simulink model "Simulink"  (R2023a)
settings: Solver=ode15s  StartTime=0.0  StopTime=10.0  RelTol=1e-3
settings Model: Creator=biom3  LastModifiedBy=biom3
settings DataIOCC: SaveOutput=off  SignalLogging=off  DSMLogging=off  SaveTime=off  ReturnWorkspaceOutputs=off

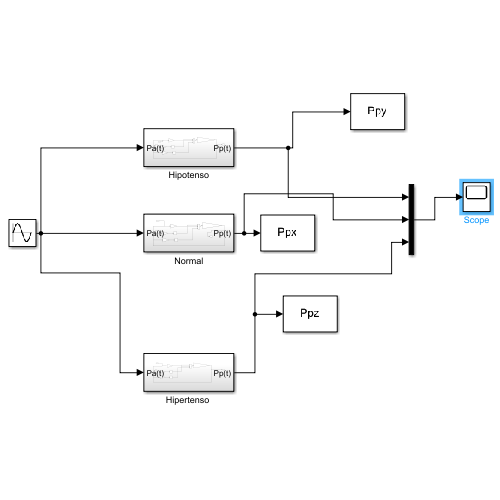
[thumbnail: Simulink's stored preview of the top-level diagram]
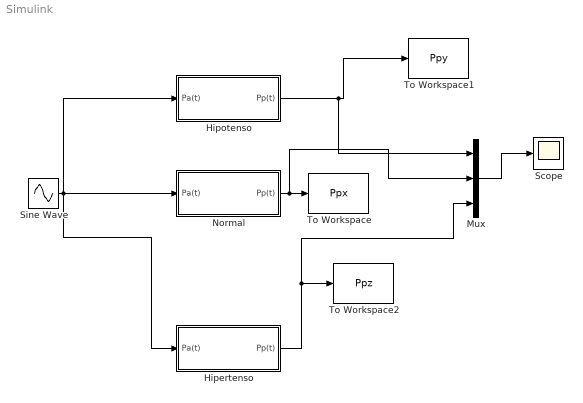
== system Simulink ==
  "Hipertenso " : Subsystem
  Hipotenso : Subsystem
  Mux : Mux  Inputs=3
  Normal : Subsystem
  Scope : Scope
  Sine Wave : Sin  Frequency=2*pi*(95/61)  SampleTime=0
  To Workspace : ToWorkspace  VariableName=Ppx  SaveFormat=Timeseries  SampleTime=-1
  To Workspace1 : ToWorkspace  VariableName=Ppy  SaveFormat=Timeseries  SampleTime=-1
  To Workspace2 : ToWorkspace  VariableName=Ppz  SaveFormat=Timeseries  SampleTime=-1
  wires:
  Mux/1 -> Scope/1
  Sine Wave/1 -> Hipotenso/1(Pa(t)), Normal/1(Pa(t)), "Hipertenso "/1(Pa(t))
  "Hipertenso "/1(Pp(t)) -> Mux/3, To Workspace2/1
  Normal/1(Pp(t)) -> Mux/2, To Workspace/1
  Hipotenso/1(Pp(t)) -> Mux/1, To Workspace1/1

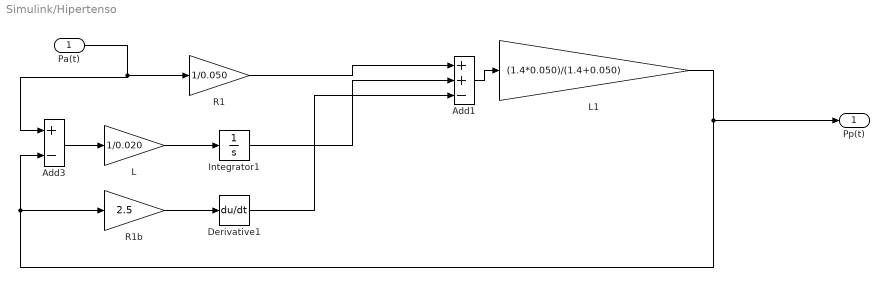
== system Simulink/Hipertenso  ==
  Pa(t) : Inport
  Add1 : Sum  Inputs=++-
  Add3 : Sum  Inputs=+-
  Derivative1 : Derivative
  Integrator1 : Integrator
  L : Gain  Gain=1/0.020
  L1 : Gain  Gain=(1.4*0.050)/(1.4+0.050)
  R1 : Gain  Gain=1/0.050
  R1b : Gain  Gain=2.5
  Pp(t) : Outport
  wires:
  Derivative1/1 -> Add1/3
  L1/1 -> Add3/2, R1b/1, Pp(t)/1
  Integrator1/1 -> Add1/2
  R1b/1 -> Derivative1/1
  R1/1 -> Add1/1
  Add1/1 -> L1/1
  Pa(t)/1 -> Add3/1, R1/1
  L/1 -> Integrator1/1
  Add3/1 -> L/1

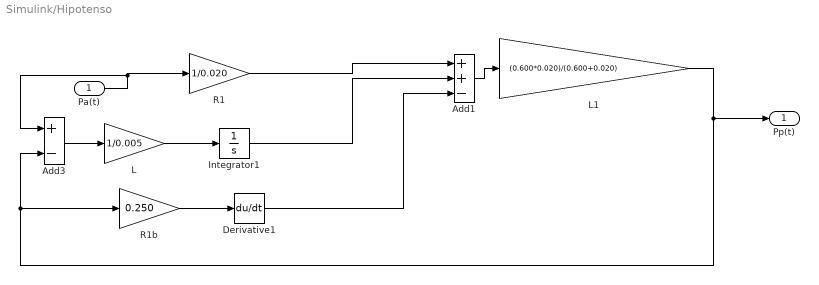
== system Simulink/Hipotenso ==
  Pa(t) : Inport
  Add1 : Sum  Inputs=++-
  Add3 : Sum  Inputs=+-
  Derivative1 : Derivative
  Integrator1 : Integrator
  L : Gain  Gain=1/0.005
  L1 : Gain  Gain=(0.600*0.020)/(0.600+0.020)
  R1 : Gain  Gain=1/0.020
  R1b : Gain  Gain=0.250
  Pp(t) : Outport
  wires:
  Derivative1/1 -> Add1/3
  L1/1 -> R1b/1, Add3/2, Pp(t)/1
  Integrator1/1 -> Add1/2
  R1b/1 -> Derivative1/1
  R1/1 -> Add1/1
  Add1/1 -> L1/1
  Pa(t)/1 -> R1/1, Add3/1
  L/1 -> Integrator1/1
  Add3/1 -> L/1

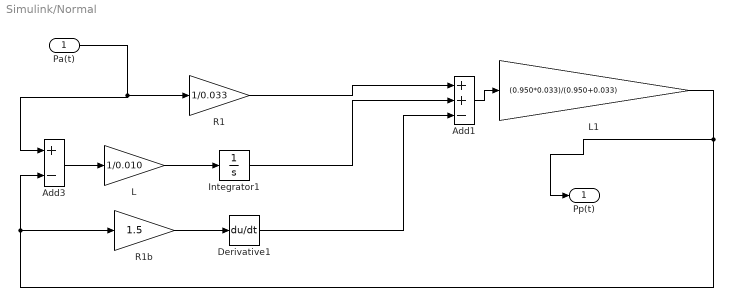
== system Simulink/Normal ==
  Pa(t) : Inport
  Add1 : Sum  Inputs=++-
  Add3 : Sum  Inputs=+-
  Derivative1 : Derivative
  Integrator1 : Integrator
  L : Gain  Gain=1/0.010
  L1 : Gain  Gain=(0.950*0.033)/(0.950+0.033)
  R1 : Gain  Gain=1/0.033
  R1b : Gain  Gain=1.5
  Pp(t) : Outport
  wires:
  Pa(t)/1 -> Add3/1, R1/1
  Add3/1 -> L/1
  R1/1 -> Add1/1
  L/1 -> Integrator1/1
  Integrator1/1 -> Add1/2
  R1b/1 -> Derivative1/1
  Derivative1/1 -> Add1/3
  Add1/1 -> L1/1
  L1/1 -> R1b/1, Add3/2, Pp(t)/1
